simulink model "TomaDatosOrden2"  (R2018b)
settings: Solver=VariableStepAuto  StartTime=0.0  StopTime=100  RelTol=1e-3
settings Model: Creator=root  LastModifiedBy=root

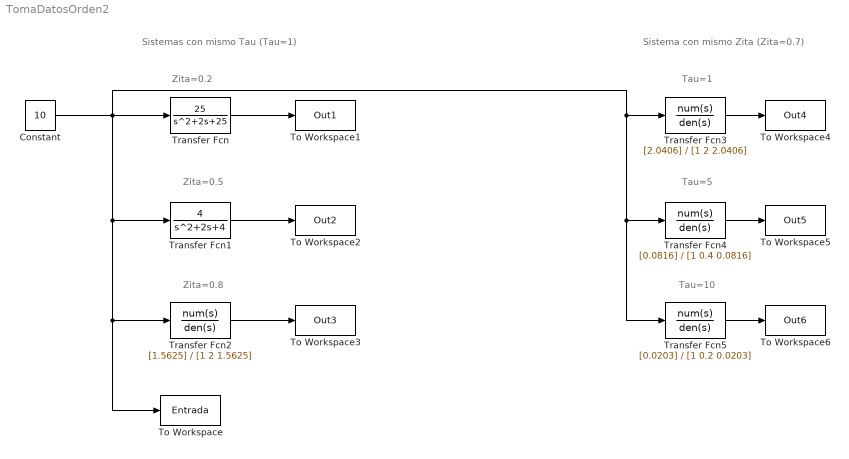
== system TomaDatosOrden2 ==
  note: Tau=10
  note: Tau=5
  note: Tau=1
  note: Zita=0.8
  note: Zita=0.5
  note: Zita=0.2
  note: Sistema con mismo Zita (Zita=0.7)
  note: Sistemas con mismo Tau (Tau=1)
  Constant : Constant  Value=10
  To Workspace : ToWorkspace  VariableName=Entrada  SampleTime=-1
  To Workspace1 : ToWorkspace  VariableName=Out1  SampleTime=0.1
  To Workspace2 : ToWorkspace  VariableName=Out2  SampleTime=0.1
  To Workspace3 : ToWorkspace  VariableName=Out3  SampleTime=0.1
  To Workspace4 : ToWorkspace  VariableName=Out4  SampleTime=0.1
  To Workspace5 : ToWorkspace  VariableName=Out5  SampleTime=0.1
  To Workspace6 : ToWorkspace  VariableName=Out6  SampleTime=0.1
  Transfer Fcn : TransferFcn  Numerator=[25]  Denominator=[1 2 25]
  Transfer Fcn1 : TransferFcn  Numerator=[4]  Denominator=[1 2 4]
  Transfer Fcn2 : TransferFcn  Numerator=[1.5625]  Denominator=[1 2 1.5625]
  Transfer Fcn3 : TransferFcn  Numerator=[2.0406]  Denominator=[1 2 2.0406]
  Transfer Fcn4 : TransferFcn  Numerator=[0.0816]  Denominator=[1 0.4 0.0816]
  Transfer Fcn5 : TransferFcn  Numerator=[0.0203]  Denominator=[1 0.2 0.0203]
  wires:
  Transfer Fcn/1 -> To Workspace1/1
  Transfer Fcn1/1 -> To Workspace2/1
  Transfer Fcn2/1 -> To Workspace3/1
  Constant/1 -> Transfer Fcn5/1, Transfer Fcn4/1, Transfer Fcn3/1, To Workspace/1, Transfer Fcn2/1, Transfer Fcn1/1, Transfer Fcn/1
  Transfer Fcn3/1 -> To Workspace4/1
  Transfer Fcn4/1 -> To Workspace5/1
  Transfer Fcn5/1 -> To Workspace6/1
